simulink model "KcontrolDeploy"  (R2021b)
settings: Solver=VariableStepAuto  StartTime=0.0  StopTime=10.0  RelTol=1e-3
undefined symbols (not defined in the file or in its folder): g, KX, KY, m_dot, m_iFuel, M_lander
libraries: slpidlib x1
settings Model: Creator=josepfamador  LastModifiedBy=josepfamador

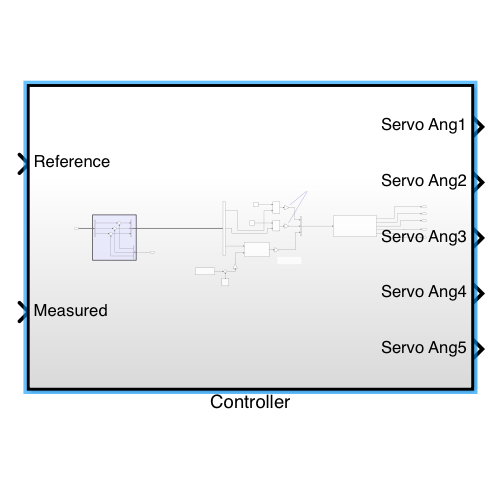
[thumbnail: Simulink's stored preview of the top-level diagram]
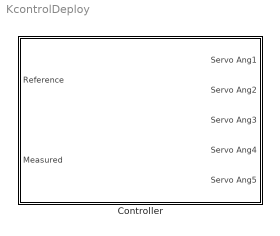
== system KcontrolDeploy ==
  Controller : Subsystem  TreatAsAtomicUnit=on

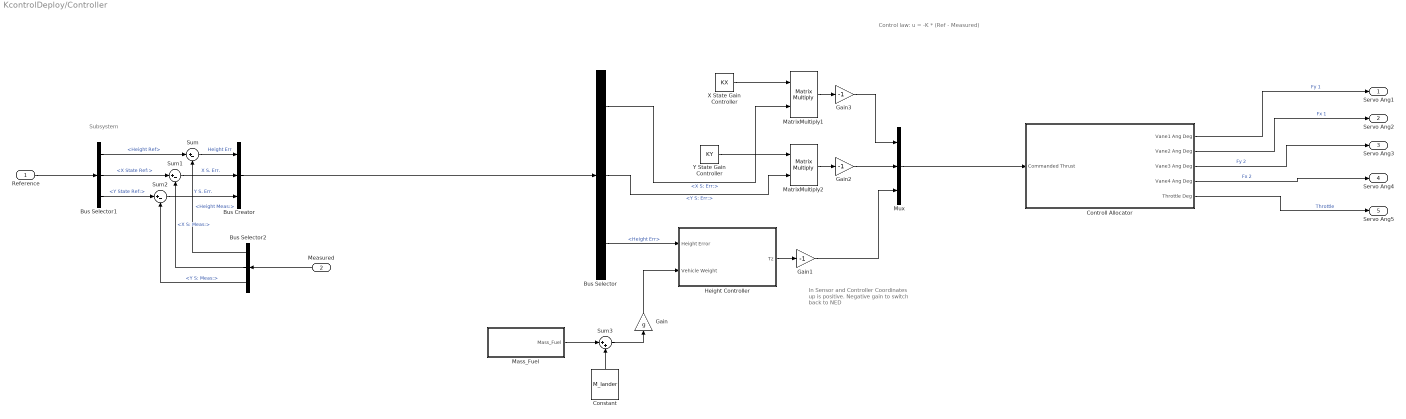
== system KcontrolDeploy/Controller ==
  note: Subsystem
  note: Control law: u = -K * (Ref - Measured)
  note: In Sensor and Controller Coordinates up is positive. Negative gain to switch back to NED
  Reference : Inport
  Measured : Inport  Port=2
  Bus Creator : BusCreator  Inputs=3
  Bus Selector : BusSelector  OutputSignals=X S: Err:,Y S: Err:,Height Err
  Bus Selector1 : BusSelector  OutputSignals=Height Ref,X State Ref:,Y State Ref:
  Bus Selector2 : BusSelector  OutputSignals=Height Meas:,X S: Meas:,Y S: Meas:
  Constant : Constant  Value=M_lander
  Controll Allocator : Subsystem
  Gain : Gain  Gain=g
  Gain1 : Gain  Gain=-1
  Gain2 : Gain  Gain=-1
  Gain3 : Gain  Gain=-1
  Height Controller : Subsystem
  Mass_Fuel : Subsystem
  MatrixMultiply1 : Product  Multiplication=Matrix(*)
  MatrixMultiply2 : Product  Multiplication=Matrix(*)
  Mux : Mux  Inputs=3
  Sum : Sum  Inputs=|+-
  Sum1 : Sum  Inputs=|+-
  Sum2 : Sum  Inputs=|+-
  Sum3 : Sum  Inputs=|++
  X State Gain Controller : Constant  Value=KX  VectorParams1D=off
  Y State Gain Controller : Constant  Value=KY  VectorParams1D=off
  Servo Ang1 : Outport
  Servo Ang2 : Outport  Port=2
  Servo Ang3 : Outport  Port=3
  Servo Ang4 : Outport  Port=4
  Servo Ang5 : Outport  Port=5
  wires:
  Height Controller/1(Tz) -> Gain1/1
  Mux/1 -> Controll Allocator/1(Commanded Thrust)
  Gain1/1 -> Mux/3
  X State Gain Controller/1 -> MatrixMultiply1/1
  Bus Selector/1 -> MatrixMultiply1/2  "<X S: Err:>"
  Y State Gain Controller/1 -> MatrixMultiply2/1
  Bus Selector/2 -> MatrixMultiply2/2  "<Y S: Err:>"
  Bus Selector/3 -> Height Controller/1(Height Error)  "<Height Err>"
  MatrixMultiply2/1 -> Gain2/1
  MatrixMultiply1/1 -> Gain3/1
  Gain2/1 -> Mux/2
  Gain3/1 -> Mux/1
  Controll Allocator/1(Vane1 Ang Deg) -> Servo Ang1/1  "Fy 1"
  Controll Allocator/2(Vane2 Ang Deg) -> Servo Ang2/1  "Fx 1"
  Controll Allocator/3(Vane3 Ang Deg) -> Servo Ang3/1  "Fy 2"
  Controll Allocator/4(Vane4 Ang Deg) -> Servo Ang4/1  "Fx 2"
  Controll Allocator/5(Throttle Deg) -> Servo Ang5/1  "Throttle"
  Reference/1 -> Bus Selector1/1
  Bus Selector2/2 -> Sum1/2  "<X S: Meas:>"
  Sum1/1 -> Bus Creator/2  "X S. Err."
  Sum2/1 -> Bus Creator/3  "Y S. Err."
  Bus Selector1/2 -> Sum1/1  "<X State Ref:>"
  Sum/1 -> Bus Creator/1  "Height Err"
  Bus Selector2/3 -> Sum2/2  "<Y S: Meas:>"
  Bus Selector1/3 -> Sum2/1  "<Y State Ref:>"
  Bus Selector1/1 -> Sum/1  "<Height Ref>"
  Bus Creator/1 -> Bus Selector/1
  Bus Selector2/1 -> Sum/2  "<Height Meas:>"
  Measured/1 -> Bus Selector2/1
  Mass_Fuel/1(Mass_Fuel) -> Sum3/1
  Constant/1 -> Sum3/2
  Sum3/1 -> Gain/1
  Gain/1 -> Height Controller/2(Vehicle Weight)

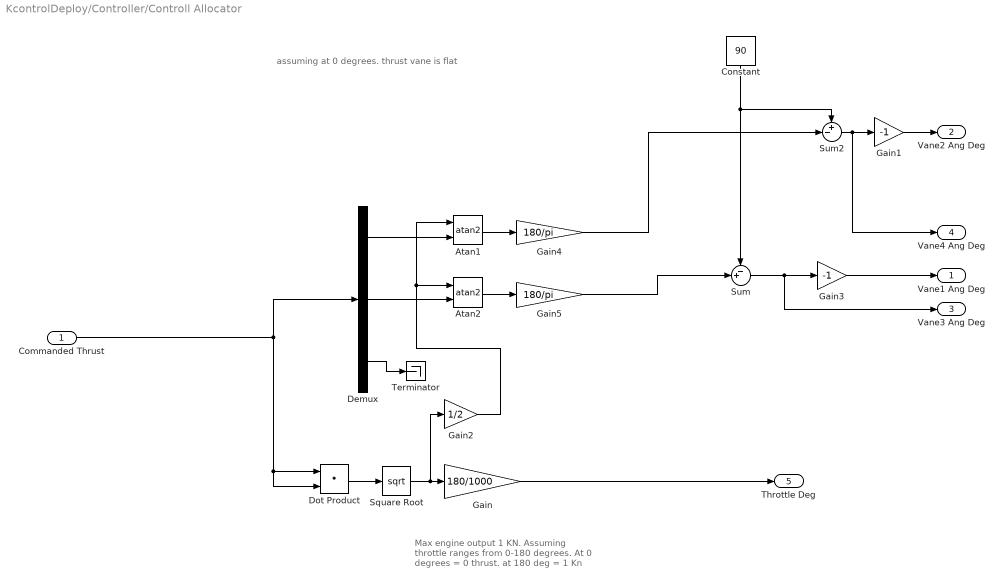
== system KcontrolDeploy/Controller/Controll Allocator ==
  note: assuming at 0 degrees. thrust vane is flat
  note: Max engine output 1 KN. Assuming throttle ranges from 0-180 degrees. At 0 degrees = 0 thrust. at 180 deg = 1 Kn
  Commanded Thrust : Inport
  Atan1 : Trigonometry  Operator=atan2
  Atan2 : Trigonometry  Operator=atan2
  Constant : Constant  Value=90
  Demux : Demux  Outputs=3
  Dot Product : DotProduct  InputSameDT=on  OutDataTypeStr=Inherit: Inherit via internal rule
  Gain : Gain  Gain=180/1000
  Gain1 : Gain  Gain=-1
  Gain2 : Gain  Gain=1/2
  Gain3 : Gain  Gain=-1
  Gain4 : Gain  Gain=180/pi
  Gain5 : Gain  Gain=180/pi
  Square Root : Sqrt  SaturateOnIntegerOverflow=on
  Sum : Sum  Inputs=-+|
  Sum2 : Sum  Inputs=+-|
  Terminator : Terminator
  Vane1 Ang Deg : Outport
  Vane2 Ang Deg : Outport  Port=2
  Vane3 Ang Deg : Outport  Port=3
  Vane4 Ang Deg : Outport  Port=4
  Throttle Deg : Outport  Port=5
  wires:
  Commanded Thrust/1 -> Demux/1, Dot Product/1, Dot Product/2
  Dot Product/1 -> Square Root/1
  Square Root/1 -> Gain2/1, Gain/1
  Gain/1 -> Throttle Deg/1
  Demux/3 -> Terminator/1
  Demux/2 -> Atan2/2
  Gain2/1 -> Atan2/1, Atan1/1
  Atan2/1 -> Gain5/1
  Constant/1 -> Sum/1, Sum2/1
  Sum/1 -> Vane3 Ang Deg/1, Gain3/1
  Demux/1 -> Atan1/2
  Atan1/1 -> Gain4/1
  Sum2/1 -> Vane4 Ang Deg/1, Gain1/1
  Gain4/1 -> Sum2/2
  Gain5/1 -> Sum/2
  Gain1/1 -> Vane2 Ang Deg/1
  Gain3/1 -> Vane1 Ang Deg/1

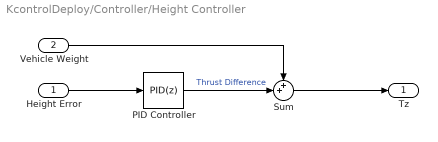
== system KcontrolDeploy/Controller/Height Controller ==
  Height Error : Inport
  Vehicle Weight : Inport  Port=2
  PID Controller : slpidlib/PID Controller  Controller=PID  Form=Parallel  TimeDomain=Discrete-time  UseExternalTs=off  SampleTime=0.1  IntegratorMethod=Forward Euler  FilterMethod=Forward Euler  ControllerParametersSource=internal  P=0.203941393902336  I=0.000548507911387826  D=13.3428538970744  UseFilter=on  N=45.4968011971303  TunerSelectOption=Transfer Function Based (PID Tuner App)  InitialConditionSource=internal  InitialConditionForIntegrator=0  InitialConditionForFilter=0  DifferentiatorICPrevScaledInput=0  ExternalReset=none  TrackingMode=off  Kt=1  LimitOutput=on  SatLimitsSource=internal  UpperSaturationLimit=500  LowerSaturationLimit=-500  LinearizeAsGain=on  AntiWindupMode=none  Kb=1  POutMin=[]  POutMax=[]  IOutMin=[]  IOutMax=[]  DOutMin=[]  DOutMax=[]  NOutMin=[]  NOutMax=[]  SumOutMin=[]  SumOutMax=[]  SaturationOutMin=[]  SaturationOutMax=[]  PParamMin=[]  PParamMax=[]  IParamMin=[]  IParamMax=[]  DParamMin=[]  DParamMax=[]  NParamMin=[]  NParamMax=[]  KbParamMin=[]  KbParamMax=[]  KtParamMin=[]  KtParamMax=[]  KbOutMin=[]  KbOutMax=[]  KtOutMin=[]  KtOutMax=[]  IntegratorOutMin=[]  IntegratorOutMax=[]  FilterOutMin=[]  FilterOutMax=[]  SumI1OutMin=[]  SumI1OutMax=[]  SumI2OutMin=[]  SumI2OutMax=[]  SumI3OutMin=[]  SumI3OutMax=[]  SumI4OutMin=[]  SumI4OutMax=[]  SumDOutMin=[]  SumDOutMax=[]  DifferentiatorOutMin=[]  DifferentiatorOutMax=[]  FilterDiffOutCoefMin=[]  FilterDiffOutCoefMax=[]  ReciprocalOutMin=[]  ReciprocalOutMax=[]  SumDenOutMin=[]  SumDenOutMax=[]  SumNumOutMin=[]  SumNumOutMax=[]  DivideOutMin=[]  DivideOutMax=[]  UdiffTsProdOutMin=[]  UdiffTsProdOutMax=[]  NTsProdOutMin=[]  NTsProdOutMax=[]  UintegralTsProdOutMin=[]  UintegralTsProdOutMax=[]  UngainTsProdOutMin=[]  UngainTsProdOutMax=[]  IntegratorContinuousStateAttributes=''  IntegratorStateMustResolveToSignalObject=off  IntegratorRTWStateStorageClass=Auto  FilterContinuousStateAttributes=''  FilterStateMustResolveToSignalObject=off  FilterRTWStateStorageClass=Auto  ParallelPVariant=InternalParameters  IdealPVariant=Disabled  IVariant=InternalParameters  DVariant=InternalParameters  IntegratorVariant=Discrete  SatVariant=Enabled  AWVariant=Passthrough  PCopyVariant=Disabled  TRVariant=Disabled  FdbkBlocksVariant=Forward  IdealPFdbkVariant=Disabled  SatFdbkVariant=Disabled  DerivativeFilterVariant=ForwardEulerFilter  NVariant=InternalParameters  NCopyVariant=Disabled  FilterICVariant=InternalICsFilter  IntegratorICVariant=InternalICs  ExternalResetVariant=Disabled  TRSumVariant=Passthrough  SumFdbkVariant=Disabled  SumVariant=Sum_PID  TsampFilterVariant=InternalTs  TsampNgainVariant=Passthrough  TsampIntegralVariant=Passthrough  ExternalSaturationOutDataTypeStr=Inherit: Same as second input
  Sum : Sum  Inputs=++|
  Tz : Outport
  wires:
  Height Error/1 -> PID Controller/1
  PID Controller/1 -> Sum/2  "Thrust Difference"
  Vehicle Weight/1 -> Sum/1
  Sum/1 -> Tz/1

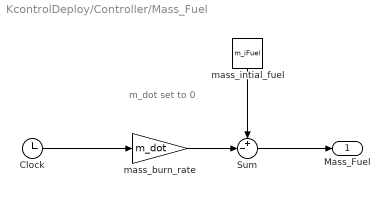
== system KcontrolDeploy/Controller/Mass_Fuel ==
  note: m_dot set to 0
  Clock : Clock
  Sum : Sum  Inputs=+-|
  mass_burn_rate : Gain  Gain=m_dot
  mass_intial_fuel : Constant  Value=m_iFuel
  Mass_Fuel : Outport
  wires:
  mass_burn_rate/1 -> Sum/2
  Sum/1 -> Mass_Fuel/1
  mass_intial_fuel/1 -> Sum/1
  Clock/1 -> mass_burn_rate/1
